simulink model "sldemo_adc_quantize"  (Simulink 6.0)
settings: Solver=VariableStepDiscrete  StartTime=0.0  StopTime=6000  FixedStep=0.1  MaxStep=0.1  RelTol=1e-3
StopFcn:
  | plot(yout.signals(1).values,double(yout.signals(2).values),'bo-'), grid, hold on, plot([0,4096],[0,4096],'g'), hold off
  | title(sprintf('Idealized A/D converter quantization algorithm \n (Zoom in close with the mouse to see behavior details)'))
  | zoom on
libraries: simulink_extras x1, simulink x1
settings Model: Creator=The MathWorks Inc.  LastModifiedBy=batserve  ExtModeAutoUpdateStatusClock=off
settings DataIOCC: ExternalInput=ustruct  LimitDataPoints=off  MaxDataPoints=5000  SaveFormat=StructureWithTime
settings OptimizationCC: BooleanDataType=off  InlineParams=on  ZeroExternalMemoryAtStartup=off  OptimizeModelRefInitCode=on  LifeSpan=1
settings DebuggingCC: CheckExecutionContextPreStartOutputMsg=on  CheckExecutionContextRuntimeOutputMsg=on
settings RTWCC: SystemTargetFile=ert.tlc  TemplateMakefile=ert_default_tmf  Description=RTW Embedded Coder (no auto configuration)  ProcessScript=ert_make_rtw_hook
settings CodeAppCC: DefineNamingRule=UpperCase  InlinedPrmAccess=Macros
settings ERTTargetCC: TargetFcnLib=iso_tfl_tmw.mat  GenFloatMathFcnCalls=ISO_C  UtilityFuncGeneration=Shared location  GenerateSampleERTMain=on  SuppressErrorStatus=on  SupportAbsoluteTime=off  SupportNonFinite=off  SupportComplex=off  InlinedParameterPlacement=NonHierarchical  RootIOFormat=Individual Arguments  ERTCustomFileTemplate=example_file_process.tlc  InitialValueSource=Model

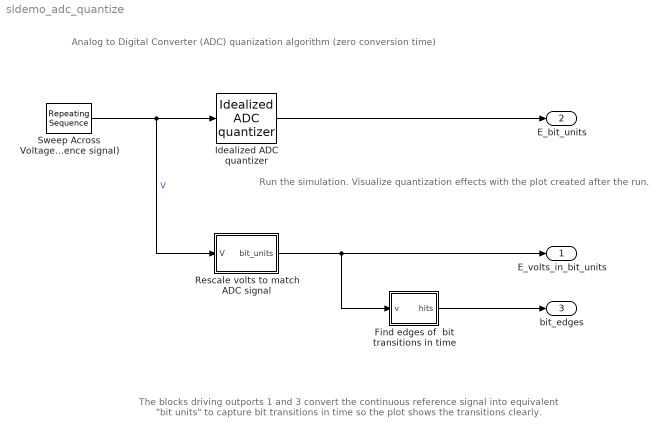
== system sldemo_adc_quantize ==
  note: Analog to Digital Converter (ADC)
      | quanization algorithm
      | (zero conversion time)
  note: The blocks driving outports 1 and 3 convert the
      | continuous reference signal into equivalent "bit units"
      | to capture bit transitions in time so the plot
      | shows the transitions clearly.
  note: Run the simulation.
      | Visualize quantization effects
      | with the plot created after the run.
  Find edges of  bit transitions in time : Subsystem  PropExecContextAcrossSSBoundary=on
  Idealized ADC quantizer : simulink_extras/Additional Discrete/Idealized ADC quantizer  NumberOfConverterBits=12  Vmin=0  Vmax=5  OutputDataType=int16  OutputNegativeValues=off
  Rescale volts to match ADC signal : Subsystem  PropExecContextAcrossSSBoundary=on
  Sweep Across Voltage Range (Reference signal) : simulink/Sources/Repeating Sequence  rep_seq_t=[0 7000]  rep_seq_y=[-0.25, 7]
  E_volts_in_bit_units : Outport
  E_bit_units : Outport  Port=2
  bit_edges : Outport  Port=3
  wires:
  Sweep Across Voltage Range (Reference signal)/1 -> Rescale volts to match ADC signal/1(V), Idealized ADC quantizer/1  "V"
  Idealized ADC quantizer/1 -> E_bit_units/1
  Rescale volts to match ADC signal/1(bit_units) -> E_volts_in_bit_units/1, Find edges of  bit transitions in time/1(v)
  Find edges of  bit transitions in time/1(hits) -> bit_edges/1

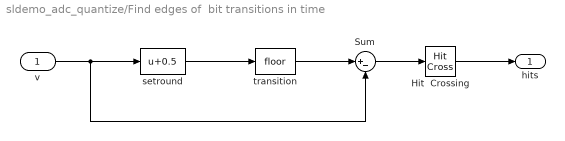
== system sldemo_adc_quantize/Find edges of  bit transitions in time ==
  v : Inport  Port=1  LatchInput=off
  Hit  Crossing : HitCross
  Sum : Sum  Inputs=|+-
  setround : Bias  Bias=0.5
  transition : Rounding
  hits : Outport
  wires:
  Sum/1 -> Hit  Crossing/1
  setround/1 -> transition/1
  transition/1 -> Sum/1
  Hit  Crossing/1 -> hits/1
  v/1 -> setround/1, Sum/2

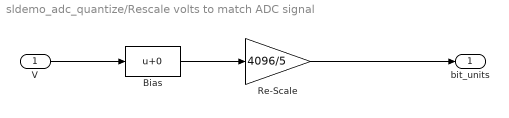
== system sldemo_adc_quantize/Rescale volts to match ADC signal ==
  V : Inport  Port=1  LatchInput=off
  Bias : Bias
  Re-Scale : Gain  Gain=4096/5
  bit_units : Outport
  wires:
  Bias/1 -> Re-Scale/1
  V/1 -> Bias/1
  Re-Scale/1 -> bit_units/1
